simulink model "FMCW_chirp_generator_RevA"  (R2021b)
settings: Solver=VariableStepAuto  StartTime=0.0  StopTime=stop_time  RelTol=1e-3
values from neighbouring files (symbols this model uses):
  chirps = obj.chirps    [Radar_revA.m]
  simulator = Simulator_revB()    [compute_sensed_targets.m]    (also in compute_sensed_values.m)
libraries: simulink x2, hdlsllib x2
settings Model: SimulationMode=accelerator  Creator=David  LastModifiedBy=David

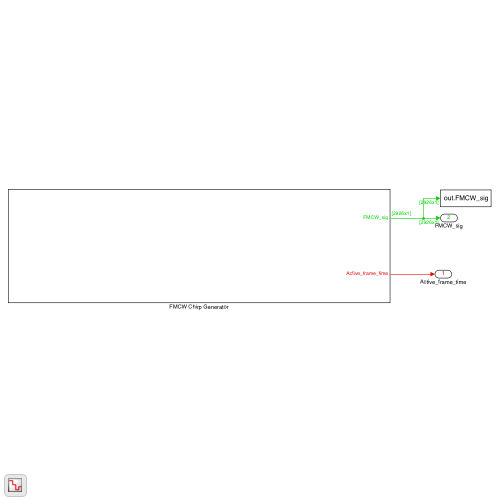
[thumbnail: Simulink's stored preview of the top-level diagram]
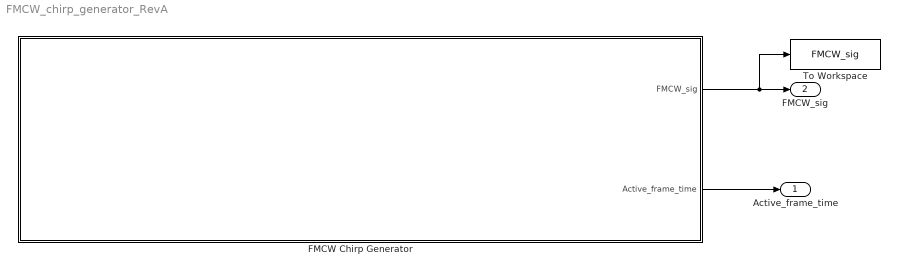
== system FMCW_chirp_generator_RevA ==
  FMCW Chirp Generator : Subsystem
  To Workspace : ToWorkspace  VariableName=FMCW_sig  SampleTime=-1
      settings: MaxDataPoints=2
  Active_frame_time : Outport
  FMCW_sig : Outport  Port=2
  wires:
  FMCW Chirp Generator/1(FMCW_sig) -> To Workspace/1, FMCW_sig/1
  FMCW Chirp Generator/2(Active_frame_time) -> Active_frame_time/1

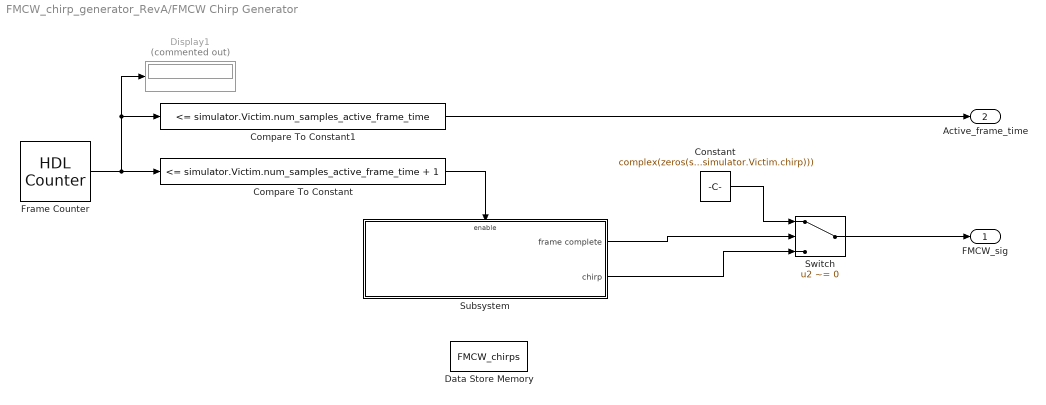
== system FMCW_chirp_generator_RevA/FMCW Chirp Generator ==
  Compare To Constant : simulink/Logic and Bit Operations/Compare To Constant  relop=<=  const=simulator.Victim.num_samples_active_frame_time + 1  OutDataTypeStr=boolean
  Compare To Constant1 : simulink/Logic and Bit Operations/Compare To Constant  relop=<=  const=simulator.Victim.num_samples_active_frame_time  OutDataTypeStr=boolean
  Constant : Constant  Value=complex(zeros(size(simulator.Victim.chirp)))  VectorParams1D=off
  Data Store Memory : DataStoreMemory  DataStoreName=FMCW_chirps  ReadBeforeWriteMsg=warning  WriteAfterWriteMsg=warning  WriteAfterReadMsg=warning  InitialValue=chirps  ShowAdditionalParam=off  OutDataTypeStr=double  Dimensions=size(chirps)
      settings: SignalType=complex
  Display1 : Display  Commented=on
  Frame Counter : hdlsllib/Sources/HDL Counter  CountType=Count limited  CountInit=1  CountStep=1  CountMax=simulator.Victim.num_samples_per_frame  CountFromType=Initial value  CountFrom=1  CountResetPort=off  CountLoadPort=off  CountEnbPort=off  CountDirPort=off  CountHitOutputPort=off  CountDataType=Unsigned  CountWordLen=32  CountFracLen=0  CountSampTime=1/simulator.Victim.FMCW_sampling_rate_Hz
  Subsystem : Subsystem
  Switch : Switch  Criteria=u2 ~= 0
  FMCW_sig : Outport
  Active_frame_time : Outport  Port=2
  wires:
  Switch/1 -> FMCW_sig/1
  Constant/1 -> Switch/1
  Subsystem/2(chirp) -> Switch/3
  Compare To Constant/1 -> Subsystem/Enable
  Frame Counter/1 -> Compare To Constant1/1, Display1/1, Compare To Constant/1
  Subsystem/1(frame complete) -> Switch/2
  Compare To Constant1/1 -> Active_frame_time/1

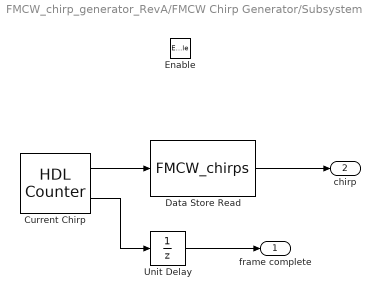
== system FMCW_chirp_generator_RevA/FMCW Chirp Generator/Subsystem ==
  Enable : EnablePort  StatesWhenEnabling=reset
  Current Chirp : hdlsllib/Sources/HDL Counter  CountType=Count limited  CountInit=1  CountStep=1  CountMax=simulator.Victim.NumChirps  CountFromType=Initial value  CountFrom=1  CountResetPort=off  CountLoadPort=off  CountEnbPort=off  CountDirPort=off  CountHitOutputPort=on  CountDataType=Signed  CountWordLen=32  CountFracLen=0  CountSampTime=simulator.Victim.ChirpCycleTime_us * 1e-6
  Data Store Read : DataStoreRead  DataStoreName=FMCW_chirps  DataStoreElements=FMCW_chirps  EnableIndexing=on  NumberOfDimensions=2  IndexOptions=Select all,Index vector (port)  Indices=1,1  OutputSizes=1,1
  Unit Delay : UnitDelay  SampleTime=-1  HasFrameUpgradeWarning=on
  frame complete : Outport
  chirp : Outport  Port=2
  wires:
  Current Chirp/1 -> Data Store Read/1
  Current Chirp/2 -> Unit Delay/1
  Data Store Read/1 -> chirp/1
  Unit Delay/1 -> frame complete/1
